simulink model "FaultLocalizationModel"  (R2024b)
settings: Solver=VariableStepAuto  StartTime=0.0  StopTime=2  RelTol=1e-3
PostLoadFcn:
  | if ~exist('stdI', 'var')
  |     stdI = 21.8182;
  | end
  | if ~exist('stdV', 'var')
  |     stdV = 5657.2;
  | end
libraries: dspai x1, dspsrcs4 x1
settings Model: Creator=pvenupra  LastModifiedBy=alial
settings DebuggingCC: ParameterPrecisionLossMsg=none

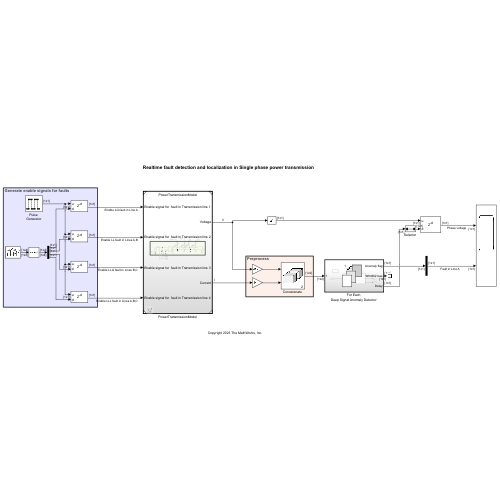
[thumbnail: Simulink's stored preview of the top-level diagram]
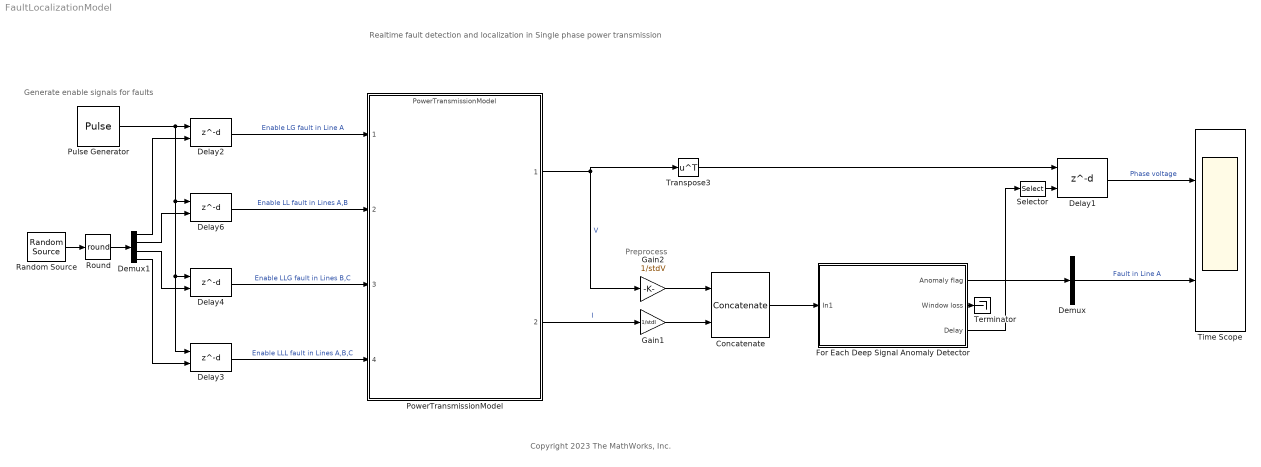
== system FaultLocalizationModel ==
  note: Copyright 2023 The MathWorks, Inc.
  note: Realtime fault detection and localization in Single phase power transmission
  note: Preprocess
  note: Generate enable signals for faults
  "Concatenate " : Concatenate  Mode=Multidimensional array  ConcatenateDimension=2
  Delay1 : Delay  DelayLengthSource=Input port  DelayLengthUpperLimit=200  DiagnosticForDelayLength=Error  RemoveDelayLengthCheckInGeneratedCode=on  InputProcessing=Columns as channels (frame based)
      settings: InputPortMap=u0,p1
  Delay{2..4,6} (4 alike) : Delay  DelayLengthSource=Input port  DelayLength=1  InputProcessing=Columns as channels (frame based)
      settings: InputPortMap=u0,p1
  Demux : Demux  Outputs=1
  Demux1 : Demux
  "For Each Deep Signal Anomaly Detector " : Subsystem  TreatAsAtomicUnit=on
  Gain1 : Gain  Gain=1/stdI
  Gain2 : Gain  Gain=1/stdV
  PowerTransmissionModel : ModelReference  ModelNameDialog=PowerTransmissionModel.slx  SimulationMode=Normal  ModelReferenceVersion=4.11
  Pulse Generator : DiscretePulseGenerator  Period=1000  PulseWidth=4  SampleTime=.025  VectorParams1D=off
  Random Source : dspsrcs4/Random Source  SrcType=Uniform  MinVal=[0 0.5 1 1.5]*40  MaxVal=[0.4 0.9 1.4 1.9]*40  MeanVal=0  VarVal=1  RepMode=Specify seed  rawSeed=0  IsInherit=off  SampTime=inf  SampFrame=1  OutComplex=Real  DataType=double  SimulateUsing=Interpreted execution
  Round : Rounding  Operator=round
  "Selector " : Selector  InputPortWidth=1  IndexOptions=Index vector (dialog)  Indices=1  OutputSizes=1
  Terminator : Terminator
  Time Scope : Scope  NumInputPorts=2
  Transpose3 : Math  Operator=transpose
  wires:
  Transpose3/1 -> Delay1/1
  Delay1/1 -> Time Scope/1  "Phase voltage"
  Gain2/1 -> "Concatenate "/1
  Gain1/1 -> "Concatenate "/2
  "Concatenate "/1 -> "For Each Deep Signal Anomaly Detector "/1(In1)
  "For Each Deep Signal Anomaly Detector "/1(Anomaly flag) -> Demux/1
  Demux/1 -> Time Scope/2  "Fault in Line A"
  "For Each Deep Signal Anomaly Detector "/3(Delay) -> "Selector "/1
  "Selector "/1 -> Delay1/2
  "For Each Deep Signal Anomaly Detector "/2(Window loss) -> Terminator/1
  PowerTransmissionModel/2 -> Gain1/1  "I"
  Demux1/4 -> Delay3/2
  Round/1 -> Demux1/1
  Delay3/1 -> PowerTransmissionModel/4  "Enable LLL fault in Lines A,B,C"
  Delay2/1 -> PowerTransmissionModel/1  "Enable LG fault in Line A"
  Demux1/1 -> Delay2/2
  Random Source/1 -> Round/1
  Pulse Generator/1 -> Delay3/1, Delay4/1, Delay6/1, Delay2/1
  Demux1/3 -> Delay4/2
  Demux1/2 -> Delay6/2
  PowerTransmissionModel/1 -> Transpose3/1, Gain2/1  "V"
  Delay6/1 -> PowerTransmissionModel/2  "Enable LL fault in Lines A,B"
  Delay4/1 -> PowerTransmissionModel/3  "Enable LLG fault in Lines B,C"

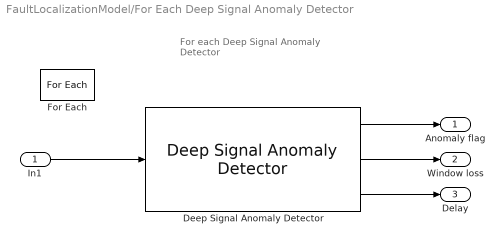
== system FaultLocalizationModel/For Each Deep Signal Anomaly Detector  ==
  note: For each
      | Deep Signal Anomaly Detector
  In1 : Inport  Partition=on  PartitionDimension=1  PartitionWidth=1  PartitionOffset=0
  "Deep Signal Anomaly Detector " : dspai/Deep Signal Anomaly Detector  DetectorMATFile=C:\Users\alial\Desktop\AUM\2024-2025\2025-Spring\osama\senior\dsp\singlePhaseFaultLocalizer.mat  ParameterSource=Read from MAT-file  WindowLength=50  OverlapLength=49  ThresholdSource=Dialog  Threshold=0.071  WindowLossAggregation=Mean  OutputDelay=on
  For Each : ForEach  DisableCoverage=on
  Anomaly flag : Outport  ConcatenationDimension=1
  Window loss : Outport  Port=2  ConcatenationDimension=1
  Delay : Outport  Port=3  ConcatenationDimension=1
  wires:
  In1/1 -> "Deep Signal Anomaly Detector "/1
  "Deep Signal Anomaly Detector "/3 -> Delay/1
  "Deep Signal Anomaly Detector "/1 -> Anomaly flag/1
  "Deep Signal Anomaly Detector "/2 -> Window loss/1
